simulink model "Flyback_Converter"  (R2023b)
settings: Solver=VariableStepAuto  StartTime=0.0  StopTime=2  RelTol=1e-3
libraries: spsVoltageMeasurementLib x3, spsSeriesRLCBranchLib x2, spsCurrentMeasurementLib x1, spsDCVoltageSourceLib x1, spsDiodeLib x1, spsLinearTransformerLib x1, spsMosfetLib x1, sps_lib x1
settings Model: Creator=vande  LastModifiedBy=vande

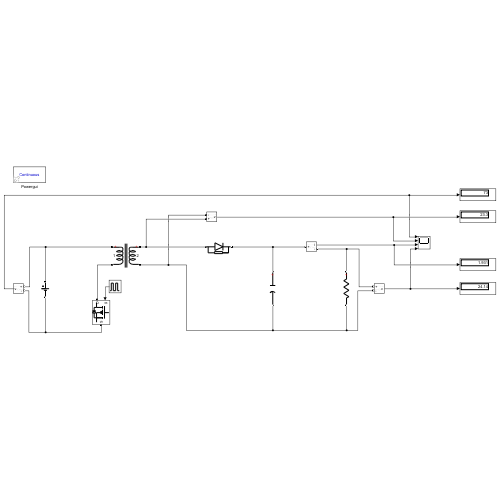
[thumbnail: Simulink's stored preview of the top-level diagram]
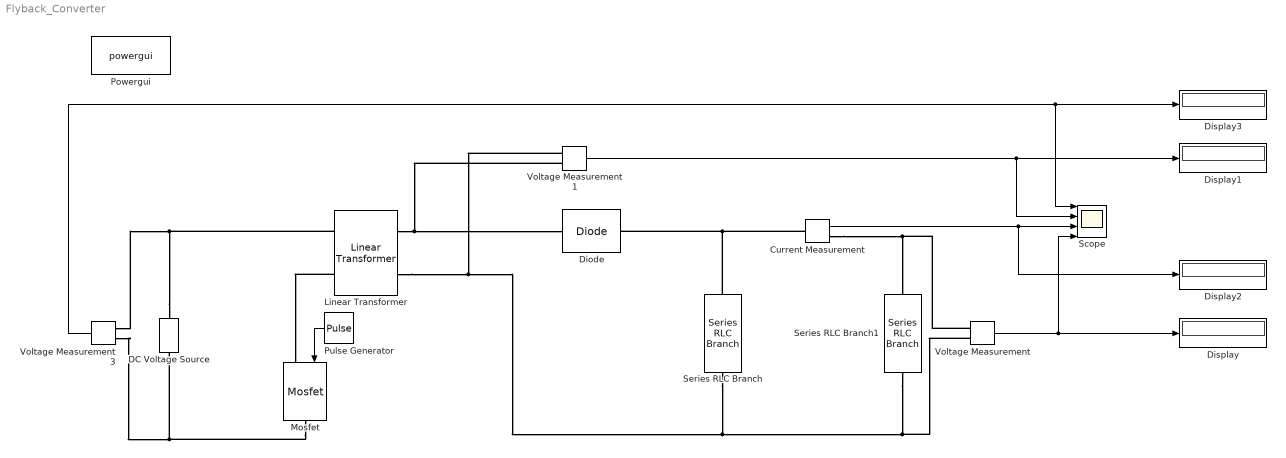
== system Flyback_Converter ==
  Current Measurement : spsCurrentMeasurementLib/Current Measurement  PhasorSimulation=off  OutputType=Complex  PSBequivalent=0
  DC Voltage Source : spsDCVoltageSourceLib/DC Voltage Source  Amplitude=73  Measurements=None
  Diode : spsDiodeLib/Diode  Ron=0.001  Lon=0  Vf=0.8  IC=0  UseSnubber=0  Rs=500  Cs=250e-9  Measurements=off
  Display{,1..3} (4 alike) : Display
  Linear Transformer : spsLinearTransformerLib/Linear Transformer  UNITS=SI  NominalPower="[ 50  50000 ]"  winding1=[73 0 0]  winding2=[25 0 0]  ThreeWindings=off  winding3=[3.15e+05 3.969e+06 505.35]  RmLm=[5.4022e+12 1.7196e+07]  Measurements=None  DataType=on
  Mosfet : spsMosfetLib/Mosfet  Ron=0.1  Lon=0  Rd=0.01  Vfd=0  IC=0  Rs=1e5  Cs=inf  Measurements=off
  Powergui : sps_lib/powergui  Priority=1  SimulationMode=Continuous  SampleTime=50e-6  frequency=60  Iterations=50  frequencyindice=0  Pbase=100e6  ErrMax=1e-4  UnitsV=kV  UnitsW=MW  buscounter=0  FunctionMessages=off  echomessages=off  EnableUseOfTLC=off  CurrentSourceSwitches=off  DisableSnubberDevices=off  DisableRonSwitches=off  DisableVfSwitches=off  DisplayEquations=off  AutomaticDiscreteSolvers=off  SolverType=Tustin/Backward Euler (TBE)  Interpol=off  ExternalGateDelay=off  methode=off  Ts=100  x0status=blocks  SPID=on  SwTol=0  HookPort=off  NonlinearTolerance=1e-4  nMaxIteration=100  ContinueOnMaxIteration=off  RestoreLinks=warning  ResistiveCurrentMeasurement=off  Frange=[0:2:500]  Ylog=off  Xlog=on  ShowGrid=off  save=off  variable=ZData  structure=0  ZoomFFT=off  StartTime=0.0  cycles=1  DisplayStyle=1  fundamental=60  FreqAxis=off  MaxFrequency=1000  frequencyindicesteady=1  RmsSteady=1  display=off
  Pulse Generator : DiscretePulseGenerator  PulseType=Time based  Amplitude=10  Period=0.00002  PulseWidth=62.50
  Scope : Scope  NumInputPorts=4
  Series RLC Branch : spsSeriesRLCBranchLib/Series RLC Branch  LConnTagsString=__new0  RConnTagsString=__new0  BranchType=C  Resistance=1  Inductance=1e-3  SetiL0=off  InitialCurrent=0  Capacitance=0.0005  Setx0=off  InitialVoltage=0  Measurements=None
  Series RLC Branch1 : spsSeriesRLCBranchLib/Series RLC Branch  LConnTagsString=__new0  RConnTagsString=__new0  BranchType=R  Resistance=12.5  Inductance=1e-3  SetiL0=off  InitialCurrent=0  Capacitance=1e-6  Setx0=off  InitialVoltage=0  Measurements=None
  Voltage Measurement : spsVoltageMeasurementLib/Voltage Measurement  PhasorSimulation=off  OutputType=Complex  PSBequivalent=0
  Voltage Measurement1 : spsVoltageMeasurementLib/Voltage Measurement  PhasorSimulation=off  OutputType=Complex  PSBequivalent=0
  Voltage Measurement3 : spsVoltageMeasurementLib/Voltage Measurement  PhasorSimulation=off  OutputType=Complex  PSBequivalent=0
  wires:
  Voltage Measurement/1 -> Display/1, Scope/4
  Pulse Generator/1 -> Mosfet/1
  Voltage Measurement3/1 -> Scope/1, Display3/1
  Voltage Measurement1/1 -> Display1/1, Scope/2
  Current Measurement/1 -> Scope/3, Display2/1
  connections:
  DC Voltage Source/RConn1 -- Voltage Measurement3/LConn1 -- Linear Transformer/LConn1
  Linear Transformer/LConn2 -- Mosfet/LConn1
  Mosfet/RConn1 -- Voltage Measurement3/LConn2 -- DC Voltage Source/LConn1
  Linear Transformer/RConn1 -- Voltage Measurement1/LConn1 -- Diode/LConn1
  Series RLC Branch1/RConn1 -- Voltage Measurement1/LConn2 -- Linear Transformer/RConn2 -- Series RLC Branch/RConn1 -- Voltage Measurement/LConn2
  Series RLC Branch/LConn1 -- Current Measurement/LConn1 -- Diode/RConn1
  Current Measurement/RConn1 -- Series RLC Branch1/LConn1 -- Voltage Measurement/LConn1
